simulink model "Filtro_velocidad"  (Simulink 9.0)
settings: Solver=ode45  StartTime=0.0  StopTime=Tsim  MaxStep=1e-3  RelTol=1e-8  EnableMultiTasking=on
values from neighbouring files (symbols this model uses):
  Tm = 0.001    [controles.m]    (also in simulaciones.m)
settings Model: Creator=Manuel G. Ortega  LastModifiedBy=Raúl  ExtModeTrigMode=oneshot  ExtModeArmWhenConnect=off
settings DataIOCC: SignalLoggingSaveFormat=ModelDataLogs
settings OptimizationCC: BooleanDataType=off  ExpressionDepthLimit=2147483647  InitFltsAndDblsToZero=on
settings DebuggingCC: SaveWithParameterizedLinksMsg=none  SignalResolutionControl=TryResolveAllWithWarning  MultiTaskDSMMsg=warning  MultiTaskCondExecSysMsg=none  FcnCallInpInsideContextMsg=warning  StateNameClashWarn=warning  StrictBusMsg=None
settings HardwareCC: TargetUnknown=on
settings GRTTargetCC: TargetFcnLib=ansi_tfl_tmw.mat  GeneratePreprocessorConditionals=Disable all  CombineOutputUpdateFcns=off  GRTInterface=on
settings ConfigComp: CovSFcnEnable=off

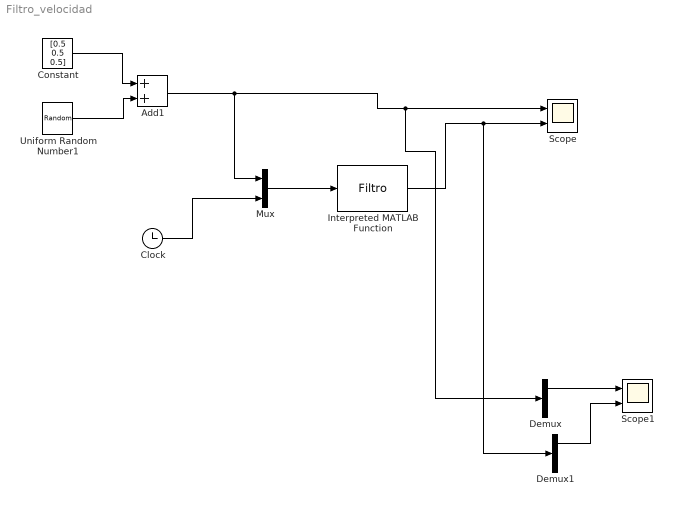
== system Filtro_velocidad ==
  Add1 : Sum
  Clock : Clock
  Constant : Constant  Value=[0.5 0.5 0.5]
  Demux : Demux  Outputs=3
  Demux1 : Demux  Outputs=3
  Interpreted MATLAB Function : MATLABFcn  MATLABFcn=Filtro  SampleTime=Tm
  Mux : Mux  Inputs=2
  Scope : Scope  NumInputPorts=2
  Scope1 : Scope  NumInputPorts=2
  Uniform Random Number1 : UniformRandomNumber  Minimum=-0.5  Maximum=0.5  SampleTime=Tm/10
  wires:
  Uniform Random Number1/1 -> Add1/2
  Constant/1 -> Add1/1
  Clock/1 -> Mux/2
  Mux/1 -> Interpreted MATLAB Function/1
  Add1/1 -> Mux/1, Demux/1, Scope/1
  Interpreted MATLAB Function/1 -> Demux1/1, Scope/2
  Demux/1 -> Scope1/1
  Demux1/1 -> Scope1/2
